simulink model "P4Simulink"  (R2024a)
settings: Solver=VariableStepAuto  StartTime=0.0  StopTime=10.0  RelTol=1e-3
InitFcn:
  | m=10;
  | r=0.05;
  | k=100;
settings Model: Creator=Becho  LastModifiedBy=Becho

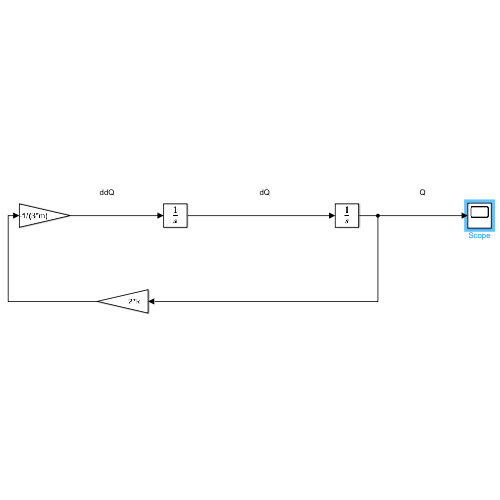
[thumbnail: Simulink's stored preview of the top-level diagram]
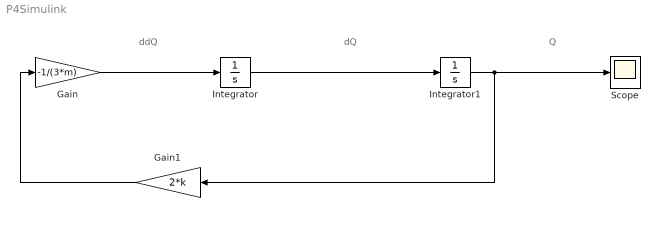
== system P4Simulink ==
  note: ddQ
  note: dQ
  note: Q
  Gain : Gain  Gain=-1/(3*m)
  Gain1 : Gain  Gain=2*k
  Integrator : Integrator  InitialCondition=2
  Integrator1 : Integrator
  Scope : Scope
  wires:
  Integrator/1 -> Integrator1/1
  Gain/1 -> Integrator/1
  Integrator1/1 -> Scope/1, Gain1/1
  Gain1/1 -> Gain/1
